simulink model "fig7_52"  (Simulink 4.00)
settings: Solver=ode23  StartTime=0.0  StopTime=5  RelTol=1e-3
settings Model: LastModifiedBy=abbas  LimitDataPoints=off  ExtModeTrigMode=oneshot  ExtModeArmWhenConnect=off  BlockReductionOpt=off

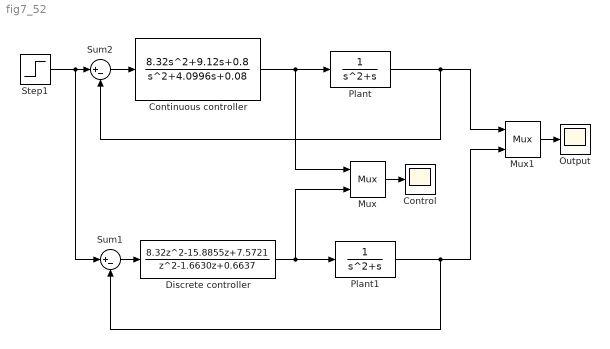
== system fig7_52 ==
  Continuous controller : TransferFcn  Numerator=[8.32 9.12 0.8]  Denominator=[1 4.0996 0.08]  Realization=auto  AbsoluteTolerance=auto
  Control : Scope
      settings: TickLabels=on  TimeRange=auto  YMin=0  YMax=2.75  SaveName=ucd  DataFormat=Array  LimitDataPoints=on  MaxDataPoints=5000
  Discrete controller : DiscreteTransferFcn  Numerator="[8.32  -15.8855 7.5721]"  Denominator=[1 -1.6630 0.6637]  SampleTime=.1  Realization=auto
  Mux : Mux  Inputs=2
      settings: DisplayOption=none
  Mux1 : Mux  Inputs=2
      settings: DisplayOption=none
  Output : Scope
      settings: TickLabels=on  TimeRange=auto  YMin=1.0035  YMax=1.01  SaveName=ycd  DataFormat=Array  LimitDataPoints=on  MaxDataPoints=5000
  Plant : TransferFcn  Numerator=[1]  Denominator="[1  1 0]"  Realization=auto  AbsoluteTolerance=auto
  Plant1 : TransferFcn  Numerator=[1]  Denominator="[1  1 0]"  Realization=auto  AbsoluteTolerance=auto
  Step1 : Step  Time=0  Before=0  After=1  SampleTime=.001
  Sum1 : Sum  Inputs=|+-  SaturateOnIntegerOverflow=off
  Sum2 : Sum  Inputs=|+-  SaturateOnIntegerOverflow=off
  wires:
  Step1/1 -> Sum2/1, Sum1/1
  Mux/1 -> Control/1
  Mux1/1 -> Output/1
  Sum1/1 -> Discrete controller/1
  Plant1/1 -> Mux1/2, Sum1/2
  Plant/1 -> Mux1/1, Sum2/2
  Sum2/1 -> Continuous controller/1
  Continuous controller/1 -> Mux/1, Plant/1
  Discrete controller/1 -> Mux/2, Plant1/1
